simulink model "sim_model_linearized"  (R2018b)
settings: Solver=ode4  StartTime=0.0  StopTime=tf  FixedStep=1e-4  RelTol=1e-3
values from neighbouring files (symbols this model uses):
  K1 = 2*K*x30^2 /x10^3    [Main.m]
  K2 = -2*K*x30/x10^2    [Main.m]
  K3 = u0/(L0*x10) - R*x30/(L0*x10) - x30*x20/x10^2    [Main.m]
  K4 = x30/x10    [Main.m]
  K5 = -R/L0 + x20/x10    (= -666.666666667)    [Main.m]
  K6 = 1/L0    (= 11.1111111111)    [Main.m]
  u0 = er    [Main.m]
  x10 = 0.03    [Main.m]
  x20 = v0    (= 0)    [Main.m]
  x30 = I0    [Main.m]
settings Model: Creator=Eduardo  LastModifiedBy=ohara

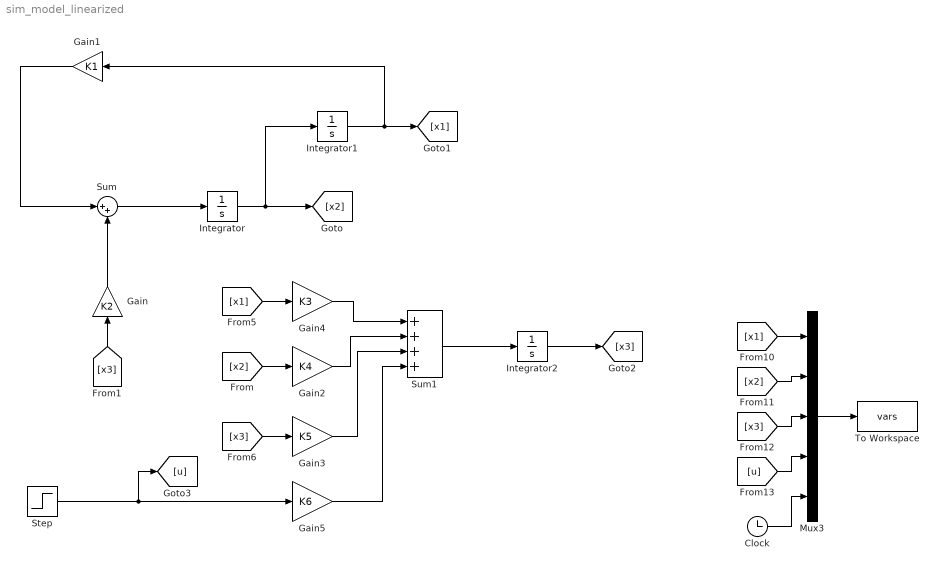
== system sim_model_linearized ==
  Clock : Clock
  Gain : Gain  Gain=K2
  Gain1 : Gain  Gain=K1
  Gain2 : Gain  Gain=K4
  Gain3 : Gain  Gain=K5
  Gain4 : Gain  Gain=K3
  Gain5 : Gain  Gain=K6
  Integrator : Integrator  InitialCondition=x20
  Integrator1 : Integrator  InitialCondition=x10
  Integrator2 : Integrator  InitialCondition=x30
  Mux3 : Mux  Inputs=5
  Step : Step  Time=0  Before=u0  After=u0  SampleTime=0
  Sum : Sum  Inputs=|++
  Sum1 : Sum  Inputs=++++
  To Workspace : ToWorkspace  VariableName=vars  SaveFormat=Timeseries  SampleTime=-1
  wires:
  Gain/1 -> Sum/2
  Sum/1 -> Integrator/1
  Integrator/1 -> Integrator1/1, [x2]
  Integrator1/1 -> Gain1/1, [x1]
  Gain1/1 -> Sum/1
  [x3] -> Gain/1
  [x2] -> Gain2/1
  Integrator2/1 -> [x3]
  Gain2/1 -> Sum1/2
  [x1] -> Gain4/1
  Gain4/1 -> Sum1/1
  [x3] -> Gain3/1
  Gain3/1 -> Sum1/3
  Sum1/1 -> Integrator2/1
  Gain5/1 -> Sum1/4
  Step/1 -> [u], Gain5/1
  Mux3/1 -> To Workspace/1
  [x1] -> Mux3/1
  [x2] -> Mux3/2
  [x3] -> Mux3/3
  [u] -> Mux3/4
  Clock/1 -> Mux3/5
